simulink model "Led5ms_SF_Topic4_Task1"  (R2019a)
settings: Solver=FixedStepDiscrete  StartTime=0.0  StopTime=Inf  RelTol=1e-3
settings Model: EnablePacing=on  Creator=Raouf  LastModifiedBy=Raouf
settings OptimizationCC: DefaultParameterBehavior=Inlined  EnhancedBackFolding=on  PassReuseOutputArgsAs=Individual arguments  OptimizeBlockOrder=speed  DifferentSizesBufferReuse=on  OptimizationCustomize=off
settings DebuggingCC: ParameterTunabilityLossMsg=error
settings SFSimCC: MATLABDynamicMemAlloc=off
settings RTWCC: SystemTargetFile=ert.tlc  GenCodeOnly=on  TemplateMakefile=ert_default_tmf  GenerateReport=on  IncludeHyperlinkInReport=on  LaunchReport=on  GenerateTraceInfo=on  GenerateTraceReport=on  GenerateTraceReportSl=on  GenerateTraceReportSf=on  GenerateTraceReportEml=on
settings CodeAppCC: ForceParamTrailComments=on  IgnoreCustomStorageClasses=off  OperatorAnnotations=on  SimulinkDataObjDesc=on  SFDataObjDesc=on  InsertBlockDesc=on
settings ERTTargetCC: TargetLangStandard=C99 (ISO)  GenerateSampleERTMain=on  InlinedParameterPlacement=NonHierarchical  ERTCustomFileTemplate=example_file_process.tlc

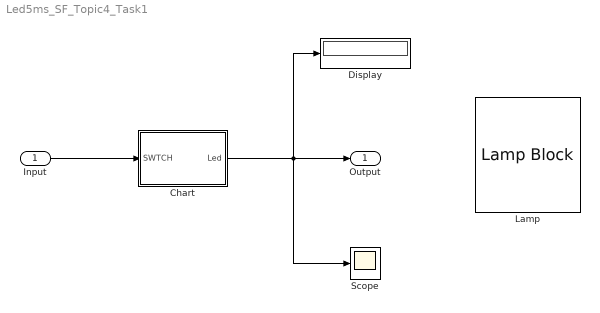
== system Led5ms_SF_Topic4_Task1 ==
  Input : Inport  OutDataTypeStr=boolean
  Chart : Stateflow chart  BlockKeywords=__PRM__SERIALIZED__DATA__:Stateflow Chart,Stateflow Diagram  TreatAsAtomicUnit=on
  Display : Display
  Lamp : LampBlock
  Scope : Scope
  Output : Outport
  wires:
  Chart/1(Led) -> Scope/1, Display/1, Output/1
  Input/1 -> Chart/1(SWTCH)

== stateflow chart Led5ms_SF_Topic4_Task1/Chart ==
  state LedOff
    en:
    Led = 0;
    du:
    Led = 0;
    exit:
    Led = 0;
  state LedOn
    en:
    Led = 1;
    du:
    Led = 1;
    exit:
    Led = 0;
  (default) -> LedOn
  LedOn -> LedOff : after(0.005,sec)
  LedOff -> LedOn : after(0.005,sec)
  data: Led output boolean; SWTCH input boolean
